simulink model "part2"  (R2019b)
settings: Solver=VariableStepAuto  StartTime=0.0  StopTime=10.0  RelTol=1e-3
settings Model: Creator=Administrateur  LastModifiedBy=Administrateur
settings SolverCC: AlgebraicLoopSolver=LineSearch

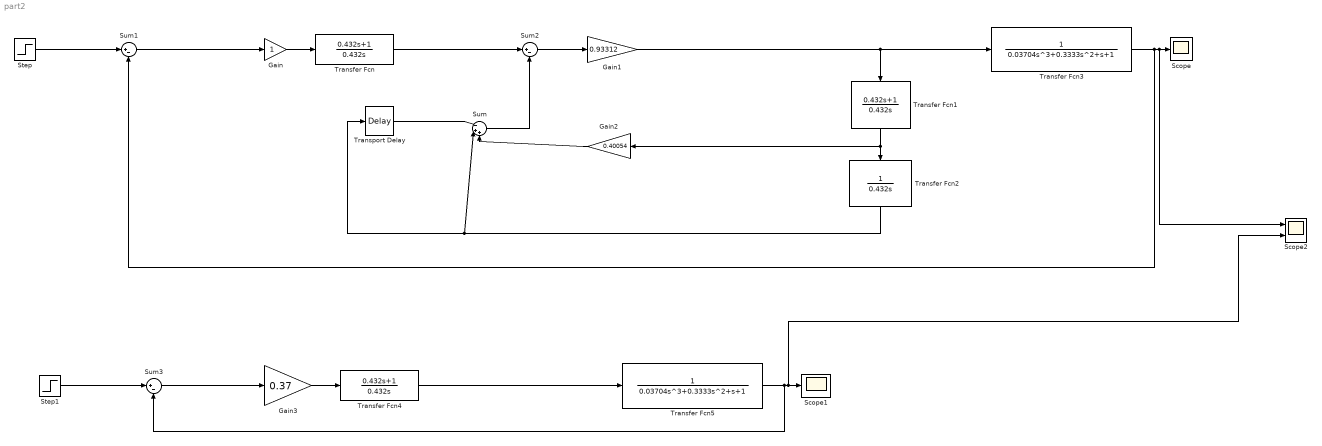
== system part2 ==
  Gain : Gain
  Gain1 : Gain  Gain=0.93312
  Gain2 : Gain  Gain=0.40054
  Gain3 : Gain  Gain=0.37
  Scope : Scope
  Scope1 : Scope
  Scope2 : Scope  NumInputPorts=2
  Step : Step  SampleTime=0
  Step1 : Step  SampleTime=0
  Sum : Sum  Inputs=|-++
  Sum1 : Sum  Inputs=|+-
  Sum2 : Sum  Inputs=|+-
  Sum3 : Sum  Inputs=|+-
  Transfer Fcn : TransferFcn  Numerator=[0.432 1]  Denominator=[0.432 0]
  Transfer Fcn1 : TransferFcn  Numerator=[0.432 1]  Denominator=[0.432 0]
  Transfer Fcn2 : TransferFcn  Denominator=[0.432 0]
  Transfer Fcn3 : TransferFcn  Denominator=[0.03704 0.3333 1 1]
  Transfer Fcn4 : TransferFcn  Numerator=[0.432 1]  Denominator=[0.432 0]
  Transfer Fcn5 : TransferFcn  Denominator=[0.03704 0.3333 1 1]
  Transport Delay : TransportDelay  DelayTime=0.3252
  wires:
  Step/1 -> Sum1/1
  Transfer Fcn3/1 -> Sum1/2, Scope2/1, Scope/1
  Transport Delay/1 -> Sum/1
  Gain1/1 -> Transfer Fcn3/1, Transfer Fcn1/1
  Transfer Fcn2/1 -> Transport Delay/1, Sum/2
  Gain/1 -> Transfer Fcn/1
  Sum2/1 -> Gain1/1
  Transfer Fcn1/1 -> Gain2/1, Transfer Fcn2/1
  Sum/1 -> Sum2/2
  Transfer Fcn/1 -> Sum2/1
  Gain2/1 -> Sum/3
  Sum1/1 -> Gain/1
  Transfer Fcn4/1 -> Transfer Fcn5/1
  Step1/1 -> Sum3/1
  Sum3/1 -> Gain3/1
  Gain3/1 -> Transfer Fcn4/1
  Transfer Fcn5/1 -> Sum3/2, Scope2/2, Scope1/1
